simulink model "Mission_Visit_2023_06_19"  (R2019a)
settings: Solver=FixedStepAuto  StartTime=0.0  StopTime=125  FixedStep=0.2  RelTol=1e-3
settings Model: Creator=anton  LastModifiedBy=anton

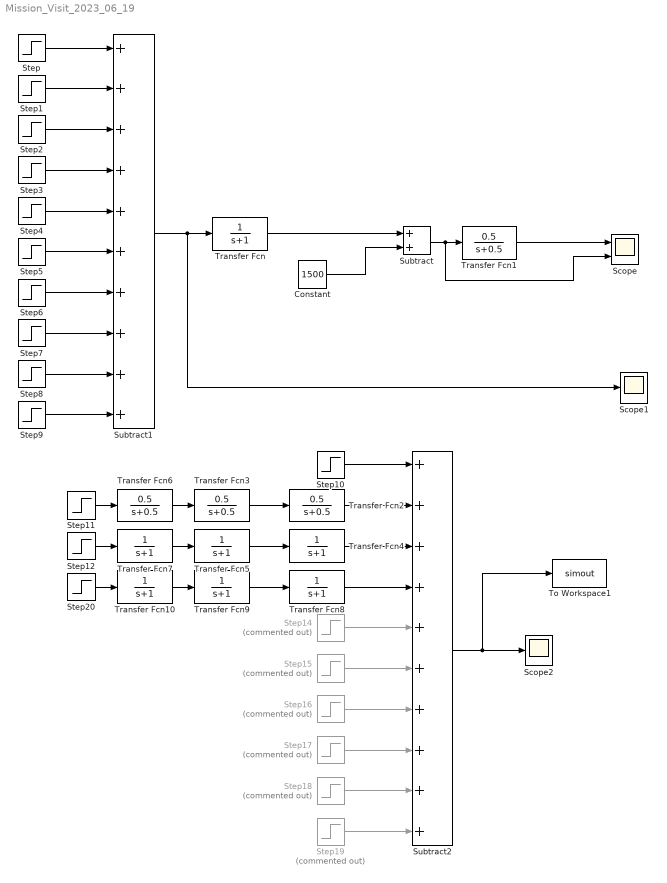
== system Mission_Visit_2023_06_19 ==
  Constant : Constant  Value=1500
  Scope : Scope  NumInputPorts=2
  Scope1 : Scope
  Scope2 : Scope
  Step : Step  After=1000  SampleTime=0
  Step1 : Step  Time=6  After=500  SampleTime=0
  Step10 : Step  Time=5  After=2000  SampleTime=0
  Step11 : Step  Time=25  After=500  SampleTime=0
  Step12 : Step  Time=75  After=-700  SampleTime=0
  Step14 : Step  Commented=on  Time=45  After=1200  SampleTime=0
  Step15 : Step  Commented=on  Time=55  After=-800  SampleTime=0
  Step16 : Step  Commented=on  Time=34  After=300  SampleTime=0
  Step17 : Step  Commented=on  Time=36  After=200  SampleTime=0
  Step18 : Step  Commented=on  Time=44  After=-900  SampleTime=0
  Step19 : Step  Commented=on  Time=50  After=1000  SampleTime=0
  Step2 : Step  Time=16  After=-500  SampleTime=0
  Step20 : Step  Time=100  After=-300  SampleTime=0
  Step3 : Step  Time=22  After=-500  SampleTime=0
  Step4 : Step  Time=24  After=-500  SampleTime=0
  Step5 : Step  Time=28  After=700  SampleTime=0
  Step6 : Step  Time=34  After=300  SampleTime=0
  Step7 : Step  Time=36  After=200  SampleTime=0
  Step8 : Step  Time=44  After=-900  SampleTime=0
  Step9 : Step  Time=50  After=1000  SampleTime=0
  Subtract : Sum
  Subtract1 : Sum  Inputs=++++++++++
  Subtract2 : Sum  Inputs=++++++++++
  To Workspace1 : ToWorkspace  VariableName=simout  SaveFormat=Timeseries  SampleTime=-1
  Transfer Fcn{,4..5,7..10} (7 alike) : TransferFcn  Numerator=1  Denominator=[1 1]
  Transfer Fcn{1..3,6} (4 alike) : TransferFcn  Numerator=0.5  Denominator=[1 0.5]
  wires:
  Transfer Fcn/1 -> Subtract/1
  Step/1 -> Subtract1/1
  Constant/1 -> Subtract/2
  Subtract/1 -> Scope/2, Transfer Fcn1/1
  Subtract1/1 -> Scope1/1, Transfer Fcn/1
  Step1/1 -> Subtract1/2
  Step2/1 -> Subtract1/3
  Step3/1 -> Subtract1/4
  Step4/1 -> Subtract1/5
  Step5/1 -> Subtract1/6
  Step6/1 -> Subtract1/7
  Step7/1 -> Subtract1/8
  Step8/1 -> Subtract1/9
  Step9/1 -> Subtract1/10
  Transfer Fcn1/1 -> Scope/1
  Step19/1 -> Subtract2/10
  Step18/1 -> Subtract2/9
  Step17/1 -> Subtract2/8
  Step16/1 -> Subtract2/7
  Step15/1 -> Subtract2/6
  Step14/1 -> Subtract2/5
  Transfer Fcn8/1 -> Subtract2/4
  Step12/1 -> Transfer Fcn7/1
  Step11/1 -> Transfer Fcn6/1
  Step10/1 -> Subtract2/1
  Subtract2/1 -> To Workspace1/1, Scope2/1
  Transfer Fcn2/1 -> Subtract2/2
  Transfer Fcn3/1 -> Transfer Fcn2/1
  Transfer Fcn4/1 -> Subtract2/3
  Transfer Fcn5/1 -> Transfer Fcn4/1
  Transfer Fcn6/1 -> Transfer Fcn3/1
  Transfer Fcn7/1 -> Transfer Fcn5/1
  Transfer Fcn10/1 -> Transfer Fcn9/1
  Transfer Fcn9/1 -> Transfer Fcn8/1
  Step20/1 -> Transfer Fcn10/1
